simulink model "BTC_OL_Harness"  (R2017b)
settings: Solver=VariableStepAuto  StartTime=0.0  StopTime=sim_time  RelTol=1e-3  EnableMultiTasking=on
settings Model: Creator=favv5g  LastModifiedBy=nctzv8
settings DataIOCC: LimitDataPoints=on
settings OptimizationCC: LifeSpan=inf
settings DebuggingCC: AllowSymbolicDim=off  SFUnexpectedBacktrackingDiag=warning  SFNoUnconditionalDefaultTransitionDiag=warning  SFExecutionAtInitializationDiag=none
settings ModelReferenceCC: PropagateSignalLabelsOutOfModel=off
settings CodeAppCC: StateflowObjectComments=on
settings GRTTargetCC: TargetLangStandard=C89/C90 (ANSI)
settings ConfigComp: CovMetricSettings=dw  CovHtmlReporting=on  CovSaveCumulativeToWorkspaceVar=on  CovSaveSingleToWorkspaceVar=on  CovExternalEMLEnable=off

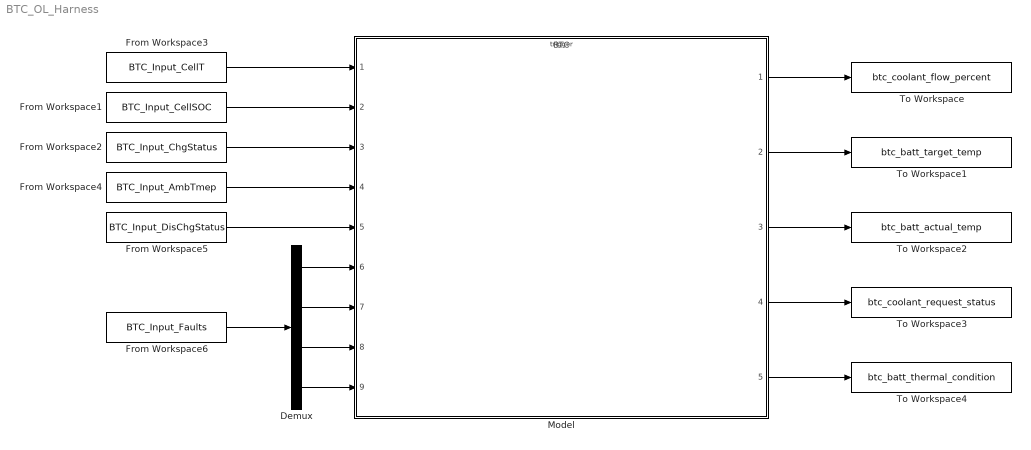
== system BTC_OL_Harness ==
  Demux : Demux
  From Workspace1 : FromWorkspace  VariableName=BTC_Input_CellSOC
  From Workspace2 : FromWorkspace  VariableName=BTC_Input_ChgStatus
  From Workspace3 : FromWorkspace  VariableName=BTC_Input_CellT
  From Workspace4 : FromWorkspace  VariableName=BTC_Input_AmbTmep
  From Workspace5 : FromWorkspace  VariableName=BTC_Input_DisChgStatus
  From Workspace6 : FromWorkspace  VariableName=BTC_Input_Faults
  Model : ModelReference  ModelNameDialog=BTC.slx  SimulationMode=Normal  ModelReferenceVersion=1.54  TriggerPortName=Trigger  TriggerPortTriggerType=function-call  TriggerPortStatesWhenEnabling=held
  To Workspace : ToWorkspace  VariableName=btc_coolant_flow_percent  SaveFormat=Timeseries  SampleTime=-1
  To Workspace1 : ToWorkspace  VariableName=btc_batt_target_temp  SaveFormat=Timeseries  SampleTime=-1
  To Workspace2 : ToWorkspace  VariableName=btc_batt_actual_temp  SaveFormat=Timeseries  SampleTime=-1
  To Workspace3 : ToWorkspace  VariableName=btc_coolant_request_status  SaveFormat=Timeseries  SampleTime=-1
  To Workspace4 : ToWorkspace  VariableName=btc_batt_thermal_condition  SaveFormat=Timeseries  SampleTime=-1
  wires:
  From Workspace3/1 -> Model/1
  From Workspace1/1 -> Model/2
  From Workspace2/1 -> Model/3
  From Workspace4/1 -> Model/4
  From Workspace5/1 -> Model/5
  From Workspace6/1 -> Demux/1
  Demux/1 -> Model/6
  Demux/2 -> Model/7
  Demux/3 -> Model/8
  Demux/4 -> Model/9
  Model/1 -> To Workspace/1
  Model/2 -> To Workspace1/1
  Model/3 -> To Workspace2/1
  Model/4 -> To Workspace3/1
  Model/5 -> To Workspace4/1
